simulink model "VVI_Pacemaker"  (R2022a)
settings: Solver=FixedStepAuto  StartTime=0.0  StopTime=10.0  FixedStep=1e-3  RelTol=1e-3  EnableMultiTasking=on
settings Model: ExtModeTrigDuration=5  Creator=yajatsharma  LastModifiedBy=yajatsharma
settings OptimizationCC: EnhancedBackFolding=on  PassReuseOutputArgsAs=Individual arguments  ZeroExternalMemoryAtStartup=off  ZeroInternalMemoryAtStartup=off  MaxStackSize=64  OptimizeBlockOrder=speed  DifferentSizesBufferReuse=on  OptimizationCustomize=off  EfficientTunableParamExpr=on
settings DebuggingCC: ParameterTunabilityLossMsg=error
settings HardwareCC: ProdBitPerPointer=32  ProdBitPerSizeT=32  ProdBitPerPtrDiffT=32  ProdLargestAtomicInteger=Long  ProdLargestAtomicFloat=Double  ProdWordSize=32  ProdHWDeviceType=ARM Compatible->ARM Cortex
settings SFSimCC: MATLABDynamicMemAlloc=off
settings RTWCC: SystemTargetFile=ert.tlc  HardwareBoard=NXP FRDM-K64F  TLCOptions="-aInlineSetEventsForThisBaseRateFcn=TLC_FALSE -aSuppressMultiTaskScheduler=TLC_FALSE  -aRateBasedStepFcn=0"  TemplateMakefile=ert_default_tmf  Toolchain=GNU Tools for ARM Embedded Processors
settings CodeAppCC: ForceParamTrailComments=on  IgnoreCustomStorageClasses=off  OperatorAnnotations=on  SimulinkDataObjDesc=on  SFDataObjDesc=on  InsertBlockDesc=on
settings ERTTargetCC: ExtModeTransport=4  ExtModeMexFile=sendToCommService

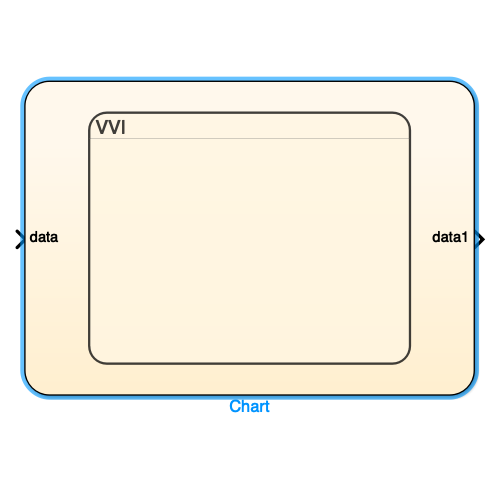
[thumbnail: Simulink's stored preview of the top-level diagram]
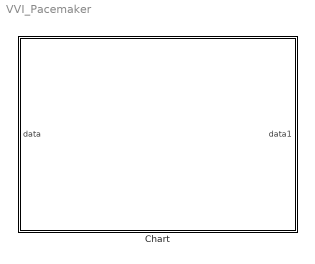
== system VVI_Pacemaker ==
  Chart : Stateflow chart  TreatAsAtomicUnit=on

== stateflow chart VVI_Pacemaker/Chart ==
  state VVI
    entry:
    Z_ATR_CTRL = 0;
    Z_VENT_CTRL =0;
    ATR_GND_CTRL = 0;
    ATR_PACE_CTRL =0;
    PACE_GND_CTRL = 1;
    PACING_REF_PWM = V_AMP;
    state DISCHARGE_C22
      entry:
      PACE_CHARGE_CTRL = 0;
      VENT_PACE_CTRL = 1;
      VENT_GND_CTRL = 0;
    state CHARGE_C22
      entry:
      VENT_PACE_CTRL = 0;
      VENT_GND_CTRL = 1;
      PACE_CHARGE_CTRL =1;
    state REFRACTORY_PERIOD
      entry:
      PACE_CHARGE_CTRL=1;
      VENT_PACE_CTRL=0;
      VENT_GND_CTRL=1;
    (default) -> CHARGE_C22
    CHARGE_C22 -> DISCHARGE_C22 : [after(VPW,msec)]
    DISCHARGE_C22 -> REFRACTORY_PERIOD : [after(VPW,msec)]
    REFRACTORY_PERIOD -> CHARGE_C22 : [after(VPW,msec)]
  data: data input int16; data1 output int16; DURATION_ON constant double =1000; LED_STATE local; DURATION_OFF constant double =1000
